simulink model "s_rotpen_bal"  (Simulink 10.0)
settings: Solver=ode1  StartTime=0.0  StopTime=10  FixedStep=0.002  RelTol=1e-3  EnableMultiTasking=on
values from neighbouring files (symbols this model uses):
  A = double(A)    [ROTPEN_ABCD_eqns_student.m]    (also in linearize.m = [0 0 1 0; 0 0 0 1; A1(1, 1:4); A1(2, 1:4)])
  B = double(B)    [ROTPEN_ABCD_eqns_student.m]    (also in linearize.m = [0; 0; A1(1, 4); A1(2, 4)])
  C = [1 0 0 0; 0 1 0 0]    [ROTPEN_ABCD_eqns_student.m]    (also in linearize.m)
  D = [0; 0]    [ROTPEN_ABCD_eqns_student.m]    (also in linearize.m)
  K = flip(K_bar)/W    [d_pole_placement_student.m]    (also in setup_rotpen.m = d_balance(A, B, zeta, wn, p3, p4))
  wcf_1 = 2 * pi * 10.0    (= 62.8318530718)    [setup_rotpen.m]
  wcf_2 = 2 * pi * 10.0    (= 62.8318530718)    [setup_rotpen.m]
libraries: simulink_extras x3
settings Model: Creator=MLevis  LastModifiedBy=isaac  ExtModeTrigDuration=10000
settings SolverCC: PositivePriorityOrder=on
settings DataIOCC: LimitDataPoints=on  SignalLoggingSaveFormat=ModelDataLogs
settings OptimizationCC: BooleanDataType=off  OptimizeBlockIOStorage=off  BufferReuse=off  GlobalBufferReuse=off  ExpressionFolding=off  ExpressionDepthLimit=2147483647  LocalBlockOutputs=off  InitFltsAndDblsToZero=on  OptimizeDataStoreBuffers=off  BusAssignmentInplaceUpdate=off
settings DebuggingCC: SaveWithParameterizedLinksMsg=none  SignalResolutionControl=TryResolveAllWithWarning  MultiTaskDSMMsg=warning  MultiTaskCondExecSysMsg=none  FcnCallInpInsideContextMsg=warning  StateNameClashWarn=warning
settings HardwareCC: TargetHWDeviceType=32-bit Generic
settings SFSimCC: SimUseLocalCustomCode=on  CustomCodeUndefinedFunction=FilterOut
settings RTWCC: Description=Quarc Win32 Target  SystemTargetFile=quarc_windows.tlc  TemplateMakefile=quarc_default_tmf  RTWUseLocalCustomCode=on
settings STFCustomTargetCC: TargetFcnLib=ansi_tfl_tmw.mat  TargetPreCompLibLocation=C:\DOCUME~1\ALLUSE~1\APPLIC~1\QUARC\lib\2007a\windows\release  CPPClassGenCompliant=on  SystemTargetFile=quarc_windows.tlc
settings GRTTargetCC: TargetFcnLib=ansi_tfl_tmw.mat  TargetPreCompLibLocation=C:\DOCUME~1\ALLUSE~1\APPLIC~1\QUARC\lib\2007a\windows\release  ParMdlRefBuildCompliant=off  CompOptLevelCompliant=off  ConcurrentExecutionCompliant=off  MatFileLogging=off  UseToolchainInfoCompliant=off  ExtMode=on  ExtModeMexFile=quarc_comm

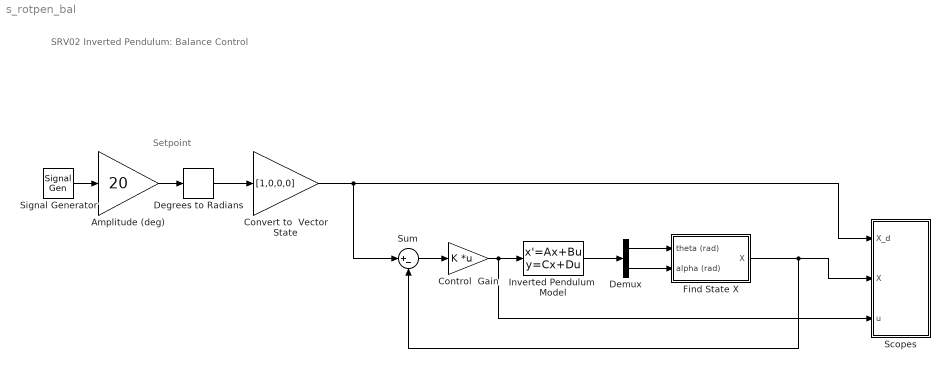
== system s_rotpen_bal ==
  note: Setpoint
  note: SRV02 Inverted Pendulum: Balance Control
  Amplitude (deg) : Gain  Gain=20  SaturateOnIntegerOverflow=on  OutDataTypeStr=Inherit: Same as input  ParamDataTypeStr=Inherit: Same as input
  Control  Gain : Gain  Gain=K  Multiplication=Matrix(K*u)
  Convert to  Vector State : Gain  Gain=[1,0,0,0]
  Degrees to Radians : simulink_extras/Transformations/Degrees to Radians
  Demux : Demux  Outputs=2
  Find State X : Subsystem
  Inverted Pendulum  Model : StateSpace  A=A  B=B  C=C  D=D  InitialCondition=0
  Scopes : Subsystem
  Signal Generator : SignalGenerator  WaveForm=square  Frequency=0.1
  Sum : Sum  Inputs=|+-
  wires:
  Amplitude (deg)/1 -> Degrees to Radians/1
  Signal Generator/1 -> Amplitude (deg)/1
  Degrees to Radians/1 -> Convert to  Vector State/1
  Convert to  Vector State/1 -> Scopes/1(X_d), Sum/1
  Find State X/1(X) -> Sum/2, Scopes/2(X)
  Sum/1 -> Control  Gain/1
  Control  Gain/1 -> Inverted Pendulum  Model/1, Scopes/3(u)
  Inverted Pendulum  Model/1 -> Demux/1
  Demux/1 -> Find State X/1(theta (rad))
  Demux/2 -> Find State X/2(alpha (rad))

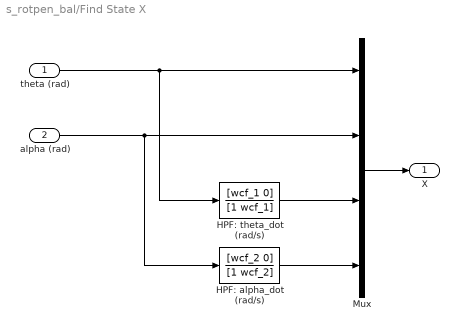
== system s_rotpen_bal/Find State X ==
  theta (rad) : Inport
  alpha (rad) : Inport  Port=2
  HPF: alpha_dot (rad/s) : TransferFcn  Numerator=[wcf_2 0]  Denominator=[1 wcf_2]
  HPF: theta_dot (rad/s) : TransferFcn  Numerator=[wcf_1 0]  Denominator=[1 wcf_1]
  Mux : Mux
  X : Outport
  wires:
  alpha (rad)/1 -> Mux/2, HPF: alpha_dot (rad/s)/1
  Mux/1 -> X/1
  theta (rad)/1 -> Mux/1, HPF: theta_dot (rad/s)/1
  HPF: theta_dot (rad/s)/1 -> Mux/3
  HPF: alpha_dot (rad/s)/1 -> Mux/4

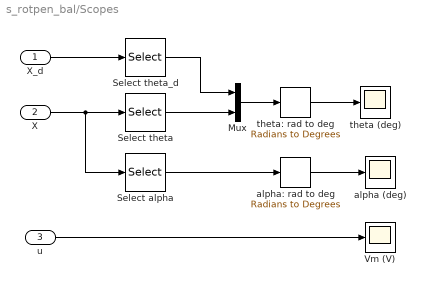
== system s_rotpen_bal/Scopes ==
  X_d : Inport
  X : Inport  Port=2
  u : Inport  Port=3
  Mux : Mux  Inputs=2
  Select alpha : Selector  InputPortWidth=4  IndexOptions=Index vector (dialog)  Indices=2  OutputSizes=[(-2)]
  Select theta : Selector  InputPortWidth=4  IndexOptions=Index vector (dialog)  Indices=1  OutputSizes=[(-2)]
  Select theta_d : Selector  InputPortWidth=4  IndexOptions=Index vector (dialog)  Indices=1  OutputSizes=[(-2)]
  Vm (V) : Scope
  alpha (deg) : Scope
  alpha: rad to deg : simulink_extras/Transformations/Radians to Degrees
  theta (deg) : Scope
  theta: rad to deg : simulink_extras/Transformations/Radians to Degrees
  wires:
  X_d/1 -> Select theta_d/1
  Select alpha/1 -> alpha: rad to deg/1
  X/1 -> Select alpha/1, Select theta/1
  Select theta_d/1 -> Mux/1
  Select theta/1 -> Mux/2
  u/1 -> Vm (V)/1
  alpha: rad to deg/1 -> alpha (deg)/1
  Mux/1 -> theta: rad to deg/1
  theta: rad to deg/1 -> theta (deg)/1
